simulink library "Suspension_Linkage_Decoupled"  (R2026a)
settings: Solver=VariableStepAuto
undefined symbols (not defined in the file): Axle1D, AxleIn, RaceFix, RaceSpin
libraries: Linkage_Decoupled x2, Suspension_Utilities x2, RollHeave_Decoupled x1, Steer_Rack x1
Description:
  | Component of Simscape Vehicle Templates Library
  | 
  | Copyright 2018-2026 The MathWorks, Inc.
settings Model: Creator=smiller  LastModifiedBy=smiller

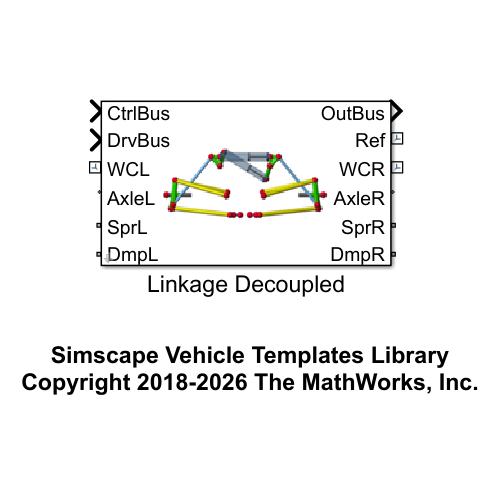
[thumbnail: Simulink's stored preview of the top-level diagram]
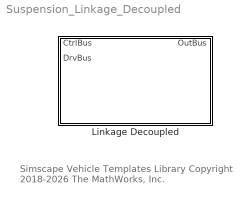
== system Suspension_Linkage_Decoupled ==
  note: Simscape Vehicle Templates Library
      | Copyright 2018-2026 The MathWorks, Inc.
  Linkage Decoupled : Subsystem  VariantControl=Linkage  mask(Linkage Decoupled){}
      mask help: Models suspension using a linkage where the stiffness and damping for the roll and heave degrees of freedom are decoupled. Includes suspension, spring and damper parts, and optional steering system. The displacement of the springs and dampers are modeled here and the forces are modeled in a separate subsystem.
      mask Display: image('sm_car_vehicle_susp_linkage_decouple_IMAGE.png');

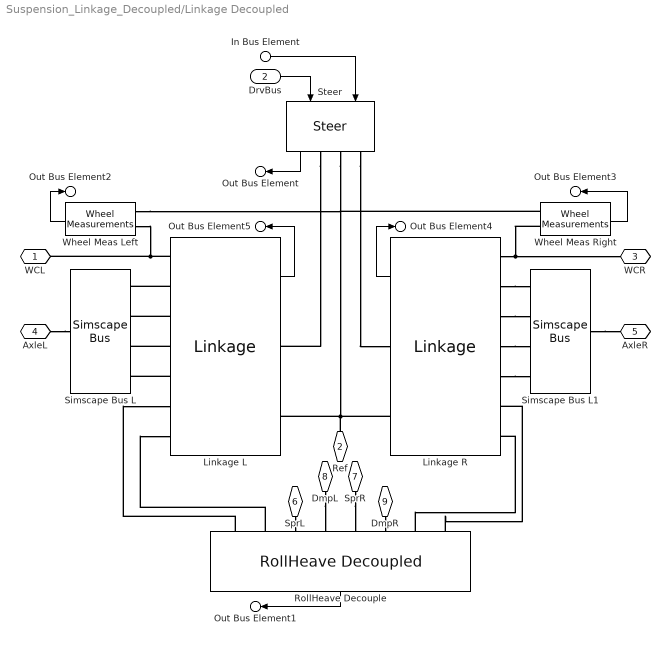
== system Suspension_Linkage_Decoupled/Linkage Decoupled ==
  In Bus Element : Inport  PortName=CtrlBus  Element=Steer
  DrvBus : Inport  Port=2
  Linkage L : Linkage_Decoupled/Linkage  VariantControl=Variant1  LabelModeActiveChoice=DWDecoupled  popup_leftRight=Left  Linkage=Susp.Linkage  InitLinkage=Init  VariantLabel=Susp.Linkage.class.Value
      settings: AttributesFormatString=%<ActiveVariant>
  Linkage R : Linkage_Decoupled/Linkage  VariantControl=Variant1  LabelModeActiveChoice=DWDecoupled  popup_leftRight=Right  Linkage=Susp.Linkage  InitLinkage=Init  VariantLabel=Susp.Linkage.class.Value
      settings: AttributesFormatString=%<ActiveVariant>
  RollHeave Decouple : RollHeave_Decoupled/RollHeave Decoupled  VariantControl=Variant1  hp_pushrod=Susp.Linkage.Pushrod.sBellcrank.Value  hp_bcr_pivot=Susp.Linkage.Bellcrank.sPivot.Value  hp_bcr_shock_heaveL=Susp.Linkage.Shock.Heave.sLeft.Value  hp_bcr_shock_heaveR=Susp.Linkage.Shock.Heave.sRight.Value  hp_bcr_shock_rollL=Susp.Linkage.Shock.Roll.sLeft.Value  hp_bcr_shock_rollR=Susp.Linkage.Shock.Roll.sRight.Value  shock_pist_mass_heave=Susp.Linkage.Shock.Heave.mPiston.Value  shock_pist_mass_roll=Susp.Linkage.Shock.Roll.mPiston.Value  shock_cyl_mass_heave=Susp.Linkage.Shock.Heave.mCylinder.Value  shock_cyl_mass_roll=Susp.Linkage.Shock.Roll.mCylinder.Value  up_lim_bumpstop_heave=Susp.Linkage.Endstop.Heave.xMax.Value  up_lim_bumpstop_roll=Susp.Linkage.Endstop.Roll.xMax.Value  low_lim_bumpstop_heave=Susp.Linkage.Endstop.Heave.xMin.Value  low_lim_bumpstop_roll=Susp.Linkage.Endstop.Roll.xMin.Value  clr_conn_shock=Visual.hp.clr  opc_conn_shock=Visual.hp.opc  size_conn_shock=Visual.hp.rad  clr_shock_cyl=Visual.Shock.cyl.clr  opc_shock_cyl=Visual.part.opc  radius_shock_cyl=Visual.Shock.cyl.rad  clr_shock_piston=Visual.Shock.piston.clr  opc_shock_piston=Visual.part.opc  clr_shock_bumpstop=Visual.Shock.bumpstop.clr  opc_shock_bumpstop=Visual.part.opc  deadvol_len_shock_cyl=Visual.Shock.dead_length  piston_len_shock=Visual.Shock.piston.len  cyl_cap_len_shock=Visual.Shock.cap.len  bumpstop_len_shock=Visual.Shock.bumpstop.len
  Simscape Bus L : SimscapeBus  HierarchyStrings=RaceSpin;RaceFix;Axle1D;AxleIn
  Simscape Bus L1 : SimscapeBus  HierarchyStrings=RaceSpin;RaceFix;Axle1D;AxleIn
  Steer : Steer_Rack/Steer  VariantControl=Steer  LabelModeActiveChoice=None  Steer=Susp.Steer  VariantLabel=Susp.Steer.class.Value
      settings: AttributesFormatString=%<ActiveVariant>
  Wheel Meas Left : Suspension_Utilities/Wheel Measurements  popup_leftRight=Left
  Wheel Meas Right : Suspension_Utilities/Wheel Measurements  popup_leftRight=Right
  WCL : PMIOPort  Side=Left
  Ref : PMIOPort  Port=2  Side=Right
  WCR : PMIOPort  Port=3  Side=Right
  AxleL : PMIOPort  Port=4  Side=Left
  AxleR : PMIOPort  Port=5  Side=Right
  SprL : PMIOPort  Port=6  Side=Left
  SprR : PMIOPort  Port=7  Side=Right
  DmpL : PMIOPort  Port=8  Side=Left
  DmpR : PMIOPort  Port=9  Side=Right
  Out Bus Element : Outport  VectorParamsAs1DForOutWhenUnconnected=off  PortName=OutBus  Element=Steer
  Out Bus Element1 : Outport  VectorParamsAs1DForOutWhenUnconnected=off  PortName=OutBus  Element=RollHeave
  Out Bus Element2 : Outport  VectorParamsAs1DForOutWhenUnconnected=off  PortName=OutBus  Element=WhlL
  Out Bus Element3 : Outport  VectorParamsAs1DForOutWhenUnconnected=off  PortName=OutBus  Element=WhlR
  Out Bus Element4 : Outport  VectorParamsAs1DForOutWhenUnconnected=off  PortName=OutBus  Element=LinkageR
  Out Bus Element5 : Outport  VectorParamsAs1DForOutWhenUnconnected=off  PortName=OutBus  Element=LinkageL
  wires:
  Wheel Meas Right/1 -> Out Bus Element3/1
  Wheel Meas Left/1 -> Out Bus Element2/1
  In Bus Element/1 -> Steer/2
  Steer/1 -> Out Bus Element/1
  DrvBus/1 -> Steer/1
  RollHeave Decouple/1 -> Out Bus Element1/1
  Linkage R/1 -> Out Bus Element4/1
  Linkage L/1 -> Out Bus Element5/1
  connections:
  RollHeave Decouple/LConn1 -- Linkage L/LConn6
  Linkage R/LConn5 -- Simscape Bus L1/LConn4
  Simscape Bus L1/RConn1 -- AxleR/RConn1
  Linkage R/LConn4 -- Simscape Bus L1/LConn3
  Linkage R/LConn3 -- Simscape Bus L1/LConn2
  Linkage R/LConn2 -- Simscape Bus L1/LConn1
  AxleL/RConn1 -- Simscape Bus L/RConn1
  Linkage L/LConn4 -- Simscape Bus L/LConn3
  Linkage L/LConn3 -- Simscape Bus L/LConn2
  Linkage L/LConn2 -- Simscape Bus L/LConn1
  Linkage L/LConn5 -- Simscape Bus L/LConn4
  Steer/RConn1 -- Linkage L/RConn1
  Wheel Meas Right/LConn2 -- Linkage R/LConn1 -- WCR/RConn1
  Wheel Meas Left/LConn2 -- Linkage L/LConn1 -- WCL/RConn1
  Steer/RConn2 -- Wheel Meas Right/LConn1 -- Wheel Meas Left/LConn1 -- Linkage R/RConn2 -- Ref/RConn1 -- Linkage L/RConn2
  Steer/RConn3 -- Linkage R/RConn1
  RollHeave Decouple/LConn2 -- Linkage L/LConn7
  RollHeave Decouple/LConn7 -- Linkage R/LConn7
  RollHeave Decouple/LConn8 -- Linkage R/LConn6
  DmpL/RConn1 -- RollHeave Decouple/LConn4
  SprL/RConn1 -- RollHeave Decouple/LConn3
  DmpR/RConn1 -- RollHeave Decouple/LConn6
  SprR/RConn1 -- RollHeave Decouple/LConn5
